simulink model "UAVIntegratedNavigationSystem"  (R2020b)
settings: Solver=FixedStepAuto  StartTime=0.0  StopTime=TFinal  FixedStep=IMUtime  RelTol=1e-3
values from neighbouring files (symbols this model uses):
  AIONtime = 1    [ModelSettings.m]
  BiasAccel = 9.81E-4    (= 0.000981)    [ModelSettings.m]
  BiasGyro = 2.424068405548E-4    (= 0.000242406840555)    [ModelSettings.m]
  CorrTimeOrientationGNSS = 1    [ModelSettings.m]
  CorrTimePositionGNSS = 1    [ModelSettings.m]
  CorrTimeVelocityGNSS = 1    [ModelSettings.m]
  delay = 1.5    [ModelSettings.m]
  e = 0.081819106    [ModelSettings.m]
  g0 = 9.780327    [ModelSettings.m]
  GNSStime = 0.2    [ModelSettings.m]
  H0 = 0.1    [ModelSettings.m]
  IMUtime = 0.01    [ModelSettings.m]
  indUAV = 2    [ModelSettings.m]
  LambdaInit = 0.6555    [ModelSettings.m]
  mass = 0.7    [ModelSettings.m]
  N = 100    [ModelSettings.m]
  PhiInit = 0.968    [ModelSettings.m]
  PitchDown = -PitchUp    (= -0.1)    [ModelSettings.m]
  PitchUp = 0.1    [ModelSettings.m]
  Ra = 6378.245    [ModelSettings.m]
  RollDown = -RollUp    (= -0.1)    [ModelSettings.m]
  RollUp = 0.1    [ModelSettings.m]
  SigmaAccel = 9.81E-4    (= 0.000981)    [ModelSettings.m]
  SigmaAION = 30    [ModelSettings.m]
  SigmaAltitudeGNSS = 3    [ModelSettings.m]
  SigmaGyro = 2.666475246102E-6    (= 2.6664752461e-06)    [ModelSettings.m]
  SigmaLaser = 5    [ModelSettings.m]
  SigmaOrientationGNSS = 0.00349    [ModelSettings.m]
  SigmaPositionGNSS = 1.5    [ModelSettings.m]
  SigmaVelocityGNSS = 0.03    [ModelSettings.m]
  SigmaVelocityUpGNSS = 0.03    [ModelSettings.m]
  U1down = 0    [ModelSettings.m]
  U1up = 4 * ForceCoeff * OmegaMax^2    (= 9.9858124)    [ModelSettings.m]
  U2down = -U2up    (= -2.4964531)    [ModelSettings.m]
  U2up = ForceCoeff * OmegaMax^2    (= 2.4964531)    [ModelSettings.m]
  U3down = -U3up    (= -2.4964531)    [ModelSettings.m]
  U3up = ForceCoeff * OmegaMax^2    (= 2.4964531)    [ModelSettings.m]
  U4down = -U4up    (= -0.2494604)    [ModelSettings.m]
  U4up = 2 * DragCoeff * OmegaMax^2    (= 0.2494604)    [ModelSettings.m]
  WEarth = 7.2921158553E-5    (= 7.2921158553e-05)    [ModelSettings.m]
undefined symbols (not defined in the file or in its folder): deg, Newton, rad, Raphson, s
libraries: simulink x11, sharedtransform x7, pid_lib x6, aerolibconvert2 x4, sharedutil x4
(part 4 of 5)

== system UAVIntegratedNavigationSystem/Блок модели динамики квадрокоптера + САУ/Полетный контроллер/Удержание положения/Row 1 ==
  Psi : Inport
  "R [1, 1]" : Subsystem
  "R [1, 2]" : Subsystem
  "R[1, 1]" : Outport
  "R[1, 2]" : Outport  Port=2
  wires:
  Psi/1 -> "R [1, 1]"/1(" Psi"), "R [1, 2]"/1(" Psi")
  "R [1, 1]"/1(R[1,1]) -> "R[1, 1]"/1
  "R [1, 2]"/1(R[1,2]) -> "R[1, 2]"/1

== system UAVIntegratedNavigationSystem/Блок модели динамики квадрокоптера + САУ/Полетный контроллер/Удержание положения/Row 2 ==
  Psi : Inport
  "R [2, 1]" : Subsystem
  "R [2, 2]" : Subsystem
  "R[2, 1]" : Outport
  "R[2, 2]" : Outport  Port=2
  wires:
  "R [2, 1]"/1(R[2,1]) -> "R[2, 1]"/1
  "R [2, 2]"/1(R[2,2]) -> "R[2, 2]"/1
  Psi/1 -> "R [2, 1]"/1(" Psi"), "R [2, 2]"/1(" Psi")

== system UAVIntegratedNavigationSystem/Блок модели динамики квадрокоптера + САУ/Упрощенная динамика БЛА /Векторы ускорений действующих сил/Ускорение силы гравитации ==
  g : Inport
  "(X, Y, Z, phi)" : Inport  Port=2
  3x3 Cross Product : sharedutil/3x3 Cross Product  aMode=aMode
      settings: SourceProductBaseCode=AE,PW,MT,UV,VE,VP
  3x3 Cross Product1 : sharedutil/3x3 Cross Product  aMode=aMode
      settings: SourceProductBaseCode=AE,PW,MT,UV,VE,VP
  Add : Sum  Inputs=+-
  Bus Selector : BusSelector  OutputSignals=X,Y,Z,phi
  Constant : Constant  Value=0
  Constant1 : Constant  Value=0
  Constant5 : Constant  Value=0
  Cos : Trigonometry  Operator=cos
  Gain : Gain  Gain=-1
  Mux : Mux  Inputs=3
  Mux1 : Mux  Inputs=3
  Mux2 : Mux  Inputs=3
  Sin2 : Trigonometry
  WEarth : Gain  Gain=WEarth
  WEarth1 : Gain  Gain=WEarth
  Вектор ускорения силы гравитации : Outport
  wires:
  Constant/1 -> Mux/1
  Constant1/1 -> Mux/3
  Gain/1 -> Mux/2
  g/1 -> Gain/1
  3x3 Cross Product/1 -> 3x3 Cross Product1/2
  Mux2/1 -> 3x3 Cross Product/2
  WEarth1/1 -> Mux1/2
  Constant5/1 -> Mux1/3
  Cos/1 -> WEarth/1
  WEarth/1 -> Mux1/1
  Sin2/1 -> WEarth1/1
  Mux1/1 -> 3x3 Cross Product1/1, 3x3 Cross Product/1
  Bus Selector/4 -> Sin2/1, Cos/1  "<phi>"
  "(X, Y, Z, phi)"/1 -> Bus Selector/1
  Mux/1 -> Add/1
  Add/1 -> Вектор ускорения силы гравитации/1
  Bus Selector/2 -> Mux2/2  "<Y>"
  Bus Selector/1 -> Mux2/1  "<X>"
  Bus Selector/3 -> Mux2/3  "<Z>"
  3x3 Cross Product1/1 -> Add/2  "Переносное ускорение"

== system UAVIntegratedNavigationSystem/Блок модели динамики квадрокоптера + САУ/Упрощенная динамика БЛА /Векторы ускорений действующих сил/Ускорение силы тяги ==
  U1 : Inport
  Pitch : Inport  Port=2
  Roll : Inport  Port=3
  Psi : Inport  Port=4
  1 / m : Gain  Gain=1/ mass
  Mux : Mux  Inputs=3
  ThrustAccX : Subsystem
  ThrustAccY : Subsystem
  ThrustAccZ : Subsystem
  Вектор ускорения силы тяги : Outport
  wires:
  U1/1 -> 1 / m/1
  Psi/1 -> ThrustAccX/4(Psi), ThrustAccZ/3(Psi)
  Pitch/1 -> ThrustAccX/2(Pitch), ThrustAccY/2(Pitch), ThrustAccZ/1(Pitch)
  1 / m/1 -> ThrustAccY/1(U1 / m), ThrustAccZ/4(U1 / m), ThrustAccX/1(U1 / m)
  Roll/1 -> ThrustAccZ/2(Roll), ThrustAccY/3(Roll), ThrustAccX/3(Roll)
  ThrustAccX/1(ThrustAccX) -> Mux/1
  ThrustAccY/1(ThrustAccY) -> Mux/2
  ThrustAccZ/1(ThrustAccZ) -> Mux/3
  Mux/1 -> Вектор ускорения силы тяги/1

== system UAVIntegratedNavigationSystem/Блок модели динамики квадрокоптера + САУ/Упрощенная динамика БЛА /Простр. движение Ц.М. БПЛА (Геогр. СК)/Координаты БПЛА (Географ. СК) ==
  Velocity : Inport
  R : Inport  Port=2
  "Север(0), Восток(0)" : Inport  Port=3
  Bus Creator : BusCreator  Inputs=5
  Demux : Demux  Outputs=2
  Demux1 : Demux  Outputs=3
  Demux2 : Demux  Outputs=2
  Integrator : Integrator  InitialCondition=PhiInit
  Integrator1 : Integrator  InitialConditionSource=external
  Integrator2 : Integrator
  Integrator3 : Integrator  InitialConditionSource=external
  Integrator4 : Integrator  InitialCondition=LambdaInit
  Product : Product
  Trigonometric Function : Trigonometry  Operator=cos
  dLambda/dt : Product  Inputs=*/
  dPhi/dt : Product  Inputs=*/
  "Coord, phi, lambda" : Outport
  wires:
  R/1 -> Demux/1
  dPhi/dt/1 -> Integrator/1
  Demux/1 -> dPhi/dt/2
  Velocity/1 -> Demux1/1
  Demux1/1 -> dPhi/dt/1, Integrator1/1
  Demux/2 -> Product/2
  Integrator1/1 -> Bus Creator/1  "X"
  Integrator2/1 -> Bus Creator/2  "Y"
  Integrator3/1 -> Bus Creator/3  "Z"
  Demux1/2 -> Integrator2/1
  Demux1/3 -> dLambda/dt/1, Integrator3/1
  Integrator/1 -> Bus Creator/4, Trigonometric Function/1  "phi"
  Trigonometric Function/1 -> Product/1
  Product/1 -> dLambda/dt/2
  dLambda/dt/1 -> Integrator4/1
  Integrator4/1 -> Bus Creator/5  "lambda"
  Bus Creator/1 -> "Coord, phi, lambda"/1
  "Север(0), Восток(0)"/1 -> Demux2/1
  Demux2/1 -> Integrator1/2
  Demux2/2 -> Integrator3/2

== system UAVIntegratedNavigationSystem/Блок модели динамики квадрокоптера + САУ/Упрощенная динамика БЛА /Простр. движение Ц.М. БПЛА (Геогр. СК)/Радиус - вектор точки местоположения Ц.М. БПЛА (phi) ==
  Phi : Inport
  Add2 : Sum  Inputs=+-
  Add3 : Sum  Inputs=+-
  Add4 : Sum
  Add5 : Sum
  Constant2 : Constant  Value=Ra
  Constant3 : Constant  Value=H0
  Constant4 : Constant
  Constant5 : Constant  Value=1.5
  Divide : Product  Inputs=*/
  Divide1 : Product  Inputs=*/
  Mux : Mux  Inputs=2
  Power : Math  Operator=pow  SaturateOnIntegerOverflow=on
  Product1 : Product
  Product2 : Product
  Sin1 : Trigonometry
  Sqrt : Sqrt  SaturateOnIntegerOverflow=on
  Square2 : Math  Operator=square  SaturateOnIntegerOverflow=on
  Square3 : Math  Operator=square  SaturateOnIntegerOverflow=on
  e1 : Constant  Value=e
  "km -> m" : Gain  Gain=1000
  "km -> m 1" : Gain  Gain=1000
  "R, м" : Outport
  wires:
  Phi/1 -> Sin1/1
  Constant2/1 -> "km -> m"/1
  Constant3/1 -> "km -> m 1"/1
  e1/1 -> Square2/1
  Square2/1 -> Product2/1, Add2/2
  Constant4/1 -> Add2/1, Add3/1
  "km -> m"/1 -> Product1/1, Divide1/1
  Add2/1 -> Product1/2
  Sin1/1 -> Square3/1
  Square3/1 -> Product2/2
  Product2/1 -> Add3/2
  Product1/1 -> Divide/1
  Divide/1 -> Add4/1
  "km -> m 1"/1 -> Add5/1, Add4/2
  Add4/1 -> Mux/1  "R1"
  Add3/1 -> Power/1, Sqrt/1
  Power/1 -> Divide/2
  Constant5/1 -> Power/2
  Mux/1 -> "R, м"/1
  Sqrt/1 -> Divide1/2
  Divide1/1 -> Add5/2
  Add5/1 -> Mux/2  "R2"

== system UAVIntegratedNavigationSystem/Блок модели динамики квадрокоптера + САУ/Упрощенная динамика БЛА /Простр. движение Ц.М. БПЛА (Геогр. СК)/Скорости БПЛА (Географ. СК) ==
  AccX : Inport
  AccY : Inport  Port=2
  AccZ : Inport  Port=3
  R : Inport  Port=4
  phi : Inport  Port=5
  Integrator : Integrator
  Integrator1 : Integrator
  Integrator2 : Integrator
  Mux : Mux  Inputs=3
  Mux1 : Mux  Inputs=3
  Mux2 : Mux  Inputs=3
  Mux3 : Mux  Inputs=2
  dVx / dt : Subsystem
  dVy / dt : Subsystem
  dVz / dt : Subsystem
  Velocity : Outport
  Относ и Кориолис ускорение : Outport  Port=2
  wires:
  Integrator/1 -> dVz / dt/5(Vx), dVy / dt/4(Vx), dVx / dt/5(Vx), Mux/1
  Integrator1/1 -> dVz / dt/3(Vy), dVx / dt/3(Vy), Mux/2
  Integrator2/1 -> Mux/3, dVz / dt/4(Vz), dVx / dt/4(Vz), dVy / dt/3(Vz)
  AccX/1 -> dVx / dt/1(AccX)
  R/1 -> dVx / dt/2(R), dVz / dt/2(R), dVy / dt/2(R)
  dVx / dt/1(dVx/dt) -> Integrator/1
  AccY/1 -> dVy / dt/1(AccY)
  dVy / dt/1(dVy/dt) -> Integrator1/1
  AccZ/1 -> dVz / dt/1(AccZ)
  dVz / dt/1(dVz/dt) -> Integrator2/1
  Mux/1 -> Velocity/1
  phi/1 -> dVx / dt/6(phi), dVy / dt/5(phi), dVz / dt/6(phi)
  dVx / dt/2(AccX относ) -> Mux1/1
  dVy / dt/2(AccY относ) -> Mux1/2
  dVz / dt/2(AccZ относ) -> Mux1/3
  dVx / dt/3(AccX кориолис) -> Mux2/1
  dVy / dt/3(AccY кориолис) -> Mux2/2
  dVz / dt/3(AccZ кориолис) -> Mux2/3
  Mux1/1 -> Mux3/1
  Mux2/1 -> Mux3/2
  Mux3/1 -> Относ и Кориолис ускорение/1

== system UAVIntegratedNavigationSystem/Блок модели динамики квадрокоптера + САУ/Упрощенная динамика БЛА /Решение уравнения Пуассона/ДУ кватернион ==
  note: p q r Q0 Q1 Q2 Q3
  state : Inport
  Bus Creator : BusCreator  Inputs=3
  Bus Selector : BusSelector  OutputSignals=wx,wy,wz
  Bus Selector1 : BusSelector  OutputSignals=wz,wy,wx
  Bus Selector2 : BusSelector  OutputSignals=wy,wz,wx
  Bus Selector3 : BusSelector  OutputSignals=wx,wz,wy
  Constant : Constant  Value=0
  Demux : Demux  Outputs=[1 1 1 4]
      settings: DisplayOption=none
  Dot Product {1..4} (4 alike) : DotProduct  InputSameDT=on  OutDataTypeStr=Inherit: Inherit via internal rule
  Gain {1..6} (6 alike) : Gain  Gain=-1  SaturateOnIntegerOverflow=on  OutDataTypeStr=Inherit: Same as input  ParamDataTypeStr=Inherit: Same as input
  Gain 7 : Gain  Gain=0.5  SaturateOnIntegerOverflow=on  OutDataTypeStr=Inherit: Same as input  ParamDataTypeStr=Inherit: Same as input
  Mux{1..4,6} (5 alike) : Mux
  d(Q)/dt : Outport
  wires:
  Mux6/1 -> Gain 7/1
  state/1 -> Demux/1
  Gain 2/1 -> Mux2/4
  Bus Selector/1 -> Gain 4/1  "<wx>"
  Mux2/1 -> Dot Product 1/2
  Mux3/1 -> Dot Product 2/2
  Mux4/1 -> Dot Product 3/2
  Demux/1 -> Bus Creator/1  "wx"
  Demux/2 -> Bus Creator/2  "wy"
  Demux/3 -> Bus Creator/3  "wz"
  Gain 5/1 -> Mux4/2
  Gain 3/1 -> Mux3/3
  Mux1/1 -> Dot Product 4/2
  Bus Creator/1 -> Bus Selector2/1, Bus Selector1/1, Bus Selector/1, Bus Selector3/1
  Constant/1 -> Mux2/1, Mux1/2, Mux3/4, Mux4/3
  Bus Selector3/3 -> Gain 1/1  "<wy>"
  Gain 4/1 -> Mux2/2
  Gain 6/1 -> Mux2/3
  Bus Selector/2 -> Gain 6/1  "<wy>"
  Bus Selector/3 -> Gain 2/1  "<wz>"
  Dot Product 2/1 -> Mux6/4
  Dot Product 3/1 -> Mux6/3
  Dot Product 4/1 -> Mux6/2
  Dot Product 1/1 -> Mux6/1
  Demux/4 -> Dot Product 3/1, Dot Product 4/1, Dot Product 1/1, Dot Product 2/1
  Gain 7/1 -> d(Q)/dt/1
  Bus Selector3/1 -> Mux1/1  "<wx>"
  Bus Selector3/2 -> Mux1/3  "<wz>"
  Gain 1/1 -> Mux1/4
  Bus Selector1/3 -> Gain 3/1  "<wx>"
  Bus Selector1/2 -> Mux3/2  "<wy>"
  Bus Selector1/1 -> Mux3/1  "<wz>"
  Bus Selector2/1 -> Mux4/1  "<wy>"
  Bus Selector2/2 -> Gain 5/1  "<wz>"
  Bus Selector2/3 -> Mux4/4  "<wx>"

== system UAVIntegratedNavigationSystem/Блок модели динамики квадрокоптера + САУ/Упрощенная динамика БЛА /Решение уравнения Пуассона/Нормирование кватерниона ==
  q : Inport  PortDimensions=4
  Product : Product  Inputs=*/  InputSameDT=on  RndMeth=Zero  SaturateOnIntegerOverflow=on  OutDataTypeStr=Inherit: Same as first input
  Square : Math  Operator=square  SignedPower=on  SaturateOnIntegerOverflow=on
  Square Root : Sqrt  Operator=signedSqrt  AlgorithmType=Newton-Raphson  SaturateOnIntegerOverflow=on
  Sum : Sum  Inputs=1  InputSameDT=on  SaturateOnIntegerOverflow=on  OutDataTypeStr=Inherit: Same as first input
  qnorm : Outport  PortDimensions=4
  wires:
  Product/1 -> qnorm/1
  Square Root/1 -> Product/2
  Square/1 -> Sum/1
  Sum/1 -> Square Root/1
  q/1 -> Product/1, Square/1

== system UAVIntegratedNavigationSystem/Показания АИОН + ЛД/Измерения АИОН + ЛД/Вектор случайных аддитивных ошибок в определении высоты местоположения БЛА/ФФ  ==
  Band-Limited White Noise1 : simulink/Sources/Band-Limited White Noise  Cov=[AIONtime]  Ts=AIONtime  seed=[23341]
  "sigma " : Gain  Gain=SigmaLaser
  Случ. погрешность ЛД по высоте : Outport
  wires:
  Band-Limited White Noise1/1 -> "sigma "/1
  "sigma "/1 -> Случ. погрешность ЛД по высоте/1

== system UAVIntegratedNavigationSystem/Показания АИОН + ЛД/Измерения АИОН + ЛД/Вектор случайных аддитивных ошибок в определении координат местоположения БЛА/ФФ  ==
  Band-Limited White Noise1 : simulink/Sources/Band-Limited White Noise  Cov=[AIONtime]  Ts=AIONtime  seed=[23341]
  sigma : Gain  Gain=SigmaAION
  Случ. погрешность АИОНпо координатам : Outport
  wires:
  sigma/1 -> Случ. погрешность АИОНпо координатам/1
  Band-Limited White Noise1/1 -> sigma/1

== system UAVIntegratedNavigationSystem/Показания приемника ГНСС/Измерения ГНСС/Вектор случайных аддитивных ошибок в определении координат местопложения БЛА/ФФ  ==
  - 1 / CorrTime : Gain  Gain=-1 / CorrTimePositionGNSS
  Add : Sum
  Band-Limited White Noise1 : simulink/Sources/Band-Limited White Noise  Cov=[GNSStime]  Ts=GNSStime  seed=[23341]
  Integrator2 : Integrator  InitialCondition=0.001
  sigma * sqrt(2 / CorrTime) : Gain  Gain=SigmaPositionGNSS * sqrt(2 / CorrTimePositionGNSS)
  Случ. погрешность ГНСС по координатам : Outport
  wires:
  Integrator2/1 -> - 1 / CorrTime/1, Случ. погрешность ГНСС по координатам/1
  Band-Limited White Noise1/1 -> sigma * sqrt(2 / CorrTime)/1
  Add/1 -> Integrator2/1
  - 1 / CorrTime/1 -> Add/1
  sigma * sqrt(2 / CorrTime)/1 -> Add/2

== system UAVIntegratedNavigationSystem/Показания приемника ГНСС/Измерения ГНСС/Вектор случайных аддитивных ошибок в определении координат местопложения БЛА/ФФ 1 ==
  - 1 / CorrTime : Gain  Gain=-1 / CorrTimePositionGNSS
  Add : Sum
  Band-Limited White Noise1 : simulink/Sources/Band-Limited White Noise  Cov=[GNSStime]  Ts=GNSStime  seed=[23341]
  Integrator2 : Integrator  InitialCondition=0.001
  sigma * sqrt(2 / CorrTime) : Gain  Gain=SigmaAltitudeGNSS * sqrt(2 / CorrTimePositionGNSS)
  Случ. погрешность ГНСС по высоте : Outport
  wires:
  Add/1 -> Integrator2/1
  Integrator2/1 -> Случ. погрешность ГНСС по высоте/1, - 1 / CorrTime/1
  sigma * sqrt(2 / CorrTime)/1 -> Add/2
  - 1 / CorrTime/1 -> Add/1
  Band-Limited White Noise1/1 -> sigma * sqrt(2 / CorrTime)/1

== system UAVIntegratedNavigationSystem/Показания приемника ГНСС/Измерения ГНСС/Вектор случайных аддитивных ошибок в определении ориентации БЛА/ФФ  ==
  - 1 / CorrTime : Gain  Gain=-1 / CorrTimeOrientationGNSS
  Add : Sum
  Band-Limited White Noise1 : simulink/Sources/Band-Limited White Noise  Cov=[GNSStime]  Ts=GNSStime  seed=[23341]
  Integrator2 : Integrator  InitialCondition=0.001
  sigma * sqrt(2 / CorrTime) : Gain  Gain=SigmaOrientationGNSS * sqrt(2 / CorrTimeOrientationGNSS)
  Случ. погрешность ГНСС по углам : Outport
  wires:
  Integrator2/1 -> - 1 / CorrTime/1, Случ. погрешность ГНСС по углам/1
  Band-Limited White Noise1/1 -> sigma * sqrt(2 / CorrTime)/1
  Add/1 -> Integrator2/1
  - 1 / CorrTime/1 -> Add/1
  sigma * sqrt(2 / CorrTime)/1 -> Add/2

== system UAVIntegratedNavigationSystem/Показания приемника ГНСС/Измерения ГНСС/Вектор случайных аддитивных ошибок в определении проекций скорости  БЛА/ФФ  ==
  - 1 / CorrTime : Gain  Gain=-1 / CorrTimeVelocityGNSS
  Add : Sum
  Band-Limited White Noise1 : simulink/Sources/Band-Limited White Noise  Cov=[GNSStime]  Ts=GNSStime  seed=[23341]
  Integrator2 : Integrator  InitialCondition=0.001
  sigma * sqrt(2 / CorrTime) : Gain  Gain=SigmaVelocityGNSS * sqrt(2 / CorrTimeVelocityGNSS)
  Случ. погрешность ГНСС по скоростям : Outport
  wires:
  Integrator2/1 -> - 1 / CorrTime/1, Случ. погрешность ГНСС по скоростям/1
  Band-Limited White Noise1/1 -> sigma * sqrt(2 / CorrTime)/1
  Add/1 -> Integrator2/1
  - 1 / CorrTime/1 -> Add/1
  sigma * sqrt(2 / CorrTime)/1 -> Add/2

== system UAVIntegratedNavigationSystem/Показания приемника ГНСС/Измерения ГНСС/Вектор случайных аддитивных ошибок в определении проекций скорости  БЛА/ФФ 1 ==
  - 1 / CorrTime : Gain  Gain=-1 / CorrTimeVelocityGNSS
  Add : Sum
  Band-Limited White Noise1 : simulink/Sources/Band-Limited White Noise  Cov=[GNSStime]  Ts=GNSStime  seed=[23341]
  Integrator2 : Integrator  InitialCondition=0.001
  sigma * sqrt(2 / CorrTime) : Gain  Gain=SigmaVelocityUpGNSS * sqrt(2 / CorrTimeVelocityGNSS)
  Случ. погрешность ГНСС по скоростям : Outport
  wires:
  Add/1 -> Integrator2/1
  Integrator2/1 -> Случ. погрешность ГНСС по скоростям/1, - 1 / CorrTime/1
  sigma * sqrt(2 / CorrTime)/1 -> Add/2
  - 1 / CorrTime/1 -> Add/1
  Band-Limited White Noise1/1 -> sigma * sqrt(2 / CorrTime)/1

== system UAVIntegratedNavigationSystem/Алгоритм ИНС /Алгоритм Навигации/Скорости БПЛА (Географ. СК)/dVx // dt/AccX Кориолис ==
  VelZ : Inport
  phi : Inport  Port=2
  2 : Constant  Value=2
  Gain : Gain  Gain=-1
  Product : Product  Inputs=4
  Trigonometric Function : Trigonometry
  WEarth : Constant  Value=WEarth
  AccX Кориолис : Outport
  wires:
  Trigonometric Function/1 -> Product/1
  Product/1 -> Gain/1
  WEarth/1 -> Product/2
  2/1 -> Product/4
  phi/1 -> Trigonometric Function/1
  VelZ/1 -> Product/3
  Gain/1 -> AccX Кориолис/1

== system UAVIntegratedNavigationSystem/Алгоритм ИНС /Алгоритм Навигации/Скорости БПЛА (Географ. СК)/dVx // dt/AccX Относительное ==
  VelX : Inport
  VelY : Inport  Port=2
  VelZ : Inport  Port=3
  R : Inport  Port=4
  phi : Inport  Port=5
  Add : Sum  Inputs=--
  Demux : Demux  Outputs=2
  Divide : Product  Inputs=*/
  Divide1 : Product  Inputs=*/
  Product1 : Product
  Product2 : Product
  Product3 : Product
  Trigonometric Function1 : Trigonometry  Operator=tan
  AccX Относительное : Outport
  wires:
  R/1 -> Demux/1
  VelZ/1 -> Product2/2, Product2/1
  Demux/2 -> Divide1/2  "R2"
  Trigonometric Function1/1 -> Product3/2
  Divide1/1 -> Product3/1
  Product2/1 -> Divide1/1
  phi/1 -> Trigonometric Function1/1
  Product3/1 -> Add/1
  Add/1 -> AccX Относительное/1
  Demux/1 -> Divide/2  "R1"
  Product1/1 -> Divide/1
  VelX/1 -> Product1/1
  VelY/1 -> Product1/2
  Divide/1 -> Add/2

== system UAVIntegratedNavigationSystem/Алгоритм ИНС /Алгоритм Навигации/Скорости БПЛА (Географ. СК)/dVy // dt/AccY Кориолис ==
  VelZ : Inport
  phi : Inport  Port=2
  2 : Constant  Value=2
  Product : Product  Inputs=4
  Trigonometric Function : Trigonometry  Operator=cos
  WEarth : Constant  Value=WEarth
  AccX Кориолис : Outport
  wires:
  Trigonometric Function/1 -> Product/1
  WEarth/1 -> Product/2
  2/1 -> Product/4
  phi/1 -> Trigonometric Function/1
  VelZ/1 -> Product/3
  Product/1 -> AccX Кориолис/1

== system UAVIntegratedNavigationSystem/Алгоритм ИНС /Алгоритм Навигации/Скорости БПЛА (Географ. СК)/dVy // dt/AccY Относительное ==
  VelX : Inport
  VelZ : Inport  Port=2
  R : Inport  Port=3
  phi : Inport  Port=4
  Add : Sum  Inputs=+-
  Demux : Demux  Outputs=2
  Divide : Product  Inputs=*/
  Divide1 : Product  Inputs=*/
  Product1 : Product
  Product2 : Product
  Product3 : Product
  Trigonometric Function1 : Trigonometry  Operator=tan
  AccY Относительное : Outport
  wires:
  R/1 -> Demux/1
  VelZ/1 -> Product2/2, Product2/1
  Product2/1 -> Divide1/1
  phi/1 -> Trigonometric Function1/1
  Divide1/1 -> Add/1
  Add/1 -> AccY Относительное/1
  Product1/1 -> Divide/1
  VelX/1 -> Product1/2, Product1/1
  Divide/1 -> Product3/1
  Demux/2 -> Divide/2  "R2"
  Demux/1 -> Divide1/2  "R1"
  Product3/1 -> Add/2
  Trigonometric Function1/1 -> Product3/2

== system UAVIntegratedNavigationSystem/Алгоритм ИНС /Алгоритм Навигации/Скорости БПЛА (Географ. СК)/dVz // dt/AccZ Кориолис ==
  VelX : Inport
  VelY : Inport  Port=2
  phi : Inport  Port=3
  2 : Constant  Value=2
  Add1 : Sum  Inputs=+-
  Gain : Gain  Gain=-1
  Product : Product  Inputs=3
  Product4 : Product
  Product5 : Product
  Trigonometric Function2 : Trigonometry  Operator=cos
  Trigonometric Function3 : Trigonometry
  WEarth : Constant  Value=WEarth
  AccZ Кориолис : Outport
  wires:
  Product5/1 -> Add1/2
  Add1/1 -> Product/3
  Product4/1 -> Add1/1
  2/1 -> Product/1
  Trigonometric Function2/1 -> Product4/2
  Trigonometric Function3/1 -> Product5/2
  WEarth/1 -> Product/2
  phi/1 -> Trigonometric Function2/1, Trigonometric Function3/1
  Product/1 -> Gain/1
  Gain/1 -> AccZ Кориолис/1
  VelY/1 -> Product4/1
  VelX/1 -> Product5/1

== system UAVIntegratedNavigationSystem/Алгоритм ИНС /Алгоритм Навигации/Скорости БПЛА (Географ. СК)/dVz // dt/AccZ Относительное ==
  VelX : Inport
  VelY : Inport  Port=2
  VelZ : Inport  Port=3
  R : Inport  Port=4
  phi : Inport  Port=5
  Add : Sum  Inputs=+-
  Demux : Demux  Outputs=2
  Divide : Product  Inputs=*/
  Divide1 : Product  Inputs=*/
  Product1 : Product
  Product2 : Product
  Product3 : Product
  Trigonometric Function1 : Trigonometry  Operator=tan
  AccZ Относительное : Outport
  wires:
  R/1 -> Demux/1
  Demux/2 -> Divide1/2  "R2"
  Trigonometric Function1/1 -> Product3/2
  Divide1/1 -> Product3/1
  Product2/1 -> Divide1/1
  phi/1 -> Trigonometric Function1/1
  Product3/1 -> Add/1
  Add/1 -> AccZ Относительное/1
  Demux/1 -> Divide/2  "R1"
  Product1/1 -> Divide/1
  Divide/1 -> Add/2
  VelY/1 -> Product1/1
  VelZ/1 -> Product2/2, Product1/2
  VelX/1 -> Product2/1

== system UAVIntegratedNavigationSystem/Алгоритм ИНС (коррекия БЧЭ)/Алгоритм Навигации/Скорости БПЛА (Географ. СК)/dVx // dt/AccX Кориолис ==
  VelZ : Inport
  phi : Inport  Port=2
  2 : Constant  Value=2
  Gain : Gain  Gain=-1
  Product : Product  Inputs=4
  Trigonometric Function : Trigonometry
  WEarth : Constant  Value=WEarth
  AccX Кориолис : Outport
  wires:
  Trigonometric Function/1 -> Product/1
  Product/1 -> Gain/1
  WEarth/1 -> Product/2
  2/1 -> Product/4
  phi/1 -> Trigonometric Function/1
  VelZ/1 -> Product/3
  Gain/1 -> AccX Кориолис/1

== system UAVIntegratedNavigationSystem/Алгоритм ИНС (коррекия БЧЭ)/Алгоритм Навигации/Скорости БПЛА (Географ. СК)/dVx // dt/AccX Относительное ==
  VelX : Inport
  VelY : Inport  Port=2
  VelZ : Inport  Port=3
  R : Inport  Port=4
  phi : Inport  Port=5
  Add : Sum  Inputs=--
  Demux : Demux  Outputs=2
  Divide : Product  Inputs=*/
  Divide1 : Product  Inputs=*/
  Product1 : Product
  Product2 : Product
  Product3 : Product
  Trigonometric Function1 : Trigonometry  Operator=tan
  AccX Относительное : Outport
  wires:
  R/1 -> Demux/1
  VelZ/1 -> Product2/2, Product2/1
  Demux/2 -> Divide1/2  "R2"
  Trigonometric Function1/1 -> Product3/2
  Divide1/1 -> Product3/1
  Product2/1 -> Divide1/1
  phi/1 -> Trigonometric Function1/1
  Product3/1 -> Add/1
  Add/1 -> AccX Относительное/1
  Demux/1 -> Divide/2  "R1"
  Product1/1 -> Divide/1
  VelX/1 -> Product1/1
  VelY/1 -> Product1/2
  Divide/1 -> Add/2

== system UAVIntegratedNavigationSystem/Алгоритм ИНС (коррекия БЧЭ)/Алгоритм Навигации/Скорости БПЛА (Географ. СК)/dVy // dt/AccY Кориолис ==
  VelZ : Inport
  phi : Inport  Port=2
  2 : Constant  Value=2
  Product : Product  Inputs=4
  Trigonometric Function : Trigonometry  Operator=cos
  WEarth : Constant  Value=WEarth
  AccX Кориолис : Outport
  wires:
  Trigonometric Function/1 -> Product/1
  WEarth/1 -> Product/2
  2/1 -> Product/4
  phi/1 -> Trigonometric Function/1
  VelZ/1 -> Product/3
  Product/1 -> AccX Кориолис/1

== system UAVIntegratedNavigationSystem/Алгоритм ИНС (коррекия БЧЭ)/Алгоритм Навигации/Скорости БПЛА (Географ. СК)/dVy // dt/AccY Относительное ==
  VelX : Inport
  VelZ : Inport  Port=2
  R : Inport  Port=3
  phi : Inport  Port=4
  Add : Sum  Inputs=+-
  Demux : Demux  Outputs=2
  Divide : Product  Inputs=*/
  Divide1 : Product  Inputs=*/
  Product1 : Product
  Product2 : Product
  Product3 : Product
  Trigonometric Function1 : Trigonometry  Operator=tan
  AccY Относительное : Outport
  wires:
  R/1 -> Demux/1
  VelZ/1 -> Product2/2, Product2/1
  Product2/1 -> Divide1/1
  phi/1 -> Trigonometric Function1/1
  Divide1/1 -> Add/1
  Add/1 -> AccY Относительное/1
  Product1/1 -> Divide/1
  VelX/1 -> Product1/2, Product1/1
  Divide/1 -> Product3/1
  Demux/2 -> Divide/2  "R2"
  Demux/1 -> Divide1/2  "R1"
  Product3/1 -> Add/2
  Trigonometric Function1/1 -> Product3/2

== system UAVIntegratedNavigationSystem/Алгоритм ИНС (коррекия БЧЭ)/Алгоритм Навигации/Скорости БПЛА (Географ. СК)/dVz // dt/AccZ Кориолис ==
  VelX : Inport
  VelY : Inport  Port=2
  phi : Inport  Port=3
  2 : Constant  Value=2
  Add1 : Sum  Inputs=+-
  Gain : Gain  Gain=-1
  Product : Product  Inputs=3
  Product4 : Product
  Product5 : Product
  Trigonometric Function2 : Trigonometry  Operator=cos
  Trigonometric Function3 : Trigonometry
  WEarth : Constant  Value=WEarth
  AccZ Кориолис : Outport
  wires:
  Product5/1 -> Add1/2
  Add1/1 -> Product/3
  Product4/1 -> Add1/1
  2/1 -> Product/1
  Trigonometric Function2/1 -> Product4/2
  Trigonometric Function3/1 -> Product5/2
  WEarth/1 -> Product/2
  phi/1 -> Trigonometric Function2/1, Trigonometric Function3/1
  Product/1 -> Gain/1
  Gain/1 -> AccZ Кориолис/1
  VelY/1 -> Product4/1
  VelX/1 -> Product5/1

== system UAVIntegratedNavigationSystem/Алгоритм ИНС (коррекия БЧЭ)/Алгоритм Навигации/Скорости БПЛА (Географ. СК)/dVz // dt/AccZ Относительное ==
  VelX : Inport
  VelY : Inport  Port=2
  VelZ : Inport  Port=3
  R : Inport  Port=4
  phi : Inport  Port=5
  Add : Sum  Inputs=+-
  Demux : Demux  Outputs=2
  Divide : Product  Inputs=*/
  Divide1 : Product  Inputs=*/
  Product1 : Product
  Product2 : Product
  Product3 : Product
  Trigonometric Function1 : Trigonometry  Operator=tan
  AccZ Относительное : Outport
  wires:
  R/1 -> Demux/1
  Demux/2 -> Divide1/2  "R2"
  Trigonometric Function1/1 -> Product3/2
  Divide1/1 -> Product3/1
  Product2/1 -> Divide1/1
  phi/1 -> Trigonometric Function1/1
  Product3/1 -> Add/1
  Add/1 -> AccZ Относительное/1
  Demux/1 -> Divide/2  "R1"
  Product1/1 -> Divide/1
  Divide/1 -> Add/2
  VelY/1 -> Product1/1
  VelZ/1 -> Product2/2, Product1/2
  VelX/1 -> Product2/1

== system UAVIntegratedNavigationSystem/Блок модели динамики квадрокоптера + САУ/Полетный контроллер/Удержание положения/Row 1/R [1, 1] ==
  " Psi" : Inport
  Cos psi 1 : Trigonometry
  R[1,1] : Outport
  wires:
  " Psi"/1 -> Cos psi 1/1
  Cos psi 1/1 -> R[1,1]/1

== system UAVIntegratedNavigationSystem/Блок модели динамики квадрокоптера + САУ/Полетный контроллер/Удержание положения/Row 1/R [1, 2] ==
  " Psi" : Inport
  Gain : Gain  Gain=-1
  Sin psi1 : Trigonometry  Operator=cos
  R[1,2] : Outport
  wires:
  " Psi"/1 -> Sin psi1/1
  Sin psi1/1 -> Gain/1
  Gain/1 -> R[1,2]/1

== system UAVIntegratedNavigationSystem/Блок модели динамики квадрокоптера + САУ/Полетный контроллер/Удержание положения/Row 2/R [2, 1] ==
  " Psi" : Inport
  Trigonometric Function : Trigonometry  Operator=cos
  R[2,1] : Outport
  wires:
  " Psi"/1 -> Trigonometric Function/1
  Trigonometric Function/1 -> R[2,1]/1

== system UAVIntegratedNavigationSystem/Блок модели динамики квадрокоптера + САУ/Полетный контроллер/Удержание положения/Row 2/R [2, 2] ==
  " Psi" : Inport
  Trigonometric Function : Trigonometry
  R[2,2] : Outport
  wires:
  " Psi"/1 -> Trigonometric Function/1
  Trigonometric Function/1 -> R[2,2]/1

== system UAVIntegratedNavigationSystem/Блок модели динамики квадрокоптера + САУ/Упрощенная динамика БЛА /Векторы ускорений действующих сил/Ускорение силы тяги/ThrustAccX ==
  U1 / m : Inport
  Pitch : Inport  Port=2
  Roll : Inport  Port=3
  Psi : Inport  Port=4
  Add : Sum  Inputs=-+
  Product : Product  Inputs=3
  Product1 : Product
  Product4 : Product
  Trigonometric Function1 : Trigonometry
  Trigonometric Function2 : Trigonometry  Operator=cos
  Trigonometric Function3 : Trigonometry  Operator=cos
  Trigonometric Function4 : Trigonometry
  Trigonometric Function5 : Trigonometry
  ThrustAccX : Outport
  wires:
  Trigonometric Function3/1 -> Product/3
  Trigonometric Function5/1 -> Product1/2
  Psi/1 -> Trigonometric Function3/1, Trigonometric Function4/1
  Trigonometric Function4/1 -> Product1/1
  Trigonometric Function2/1 -> Product/2
  Add/1 -> Product4/2
  Roll/1 -> Trigonometric Function5/1, Trigonometric Function2/1
  Product/1 -> Add/1
  Trigonometric Function1/1 -> Product/1
  Product1/1 -> Add/2
  Product4/1 -> ThrustAccX/1
  U1 / m/1 -> Product4/1
  Pitch/1 -> Trigonometric Function1/1

== system UAVIntegratedNavigationSystem/Блок модели динамики квадрокоптера + САУ/Упрощенная динамика БЛА /Векторы ускорений действующих сил/Ускорение силы тяги/ThrustAccY ==
  U1 / m : Inport
  Pitch : Inport  Port=2
  Roll : Inport  Port=3
  Product : Product
  Product1 : Product
  Trigonometric Function : Trigonometry  Operator=cos
  Trigonometric Function1 : Trigonometry  Operator=cos
  ThrustAccY : Outport
  wires:
  Trigonometric Function1/1 -> Product/2
  Pitch/1 -> Trigonometric Function/1
  Product/1 -> Product1/2
  Trigonometric Function/1 -> Product/1
  Roll/1 -> Trigonometric Function1/1
  U1 / m/1 -> Product1/1
  Product1/1 -> ThrustAccY/1

== system UAVIntegratedNavigationSystem/Блок модели динамики квадрокоптера + САУ/Упрощенная динамика БЛА /Векторы ускорений действующих сил/Ускорение силы тяги/ThrustAccZ ==
  Pitch : Inport
  Roll : Inport  Port=2
  Psi : Inport  Port=3
  U1 / m : Inport  Port=4
  Add : Sum
  Product1 : Product
  Product2 : Product  Inputs=3
  Product4 : Product
  Trigonometric Function1 : Trigonometry  Operator=cos
  Trigonometric Function2 : Trigonometry
  Trigonometric Function3 : Trigonometry
  Trigonometric Function4 : Trigonometry  Operator=cos
  Trigonometric Function5 : Trigonometry
  ThrustAccZ : Outport
  wires:
  Trigonometric Function3/1 -> Product2/3
  Trigonometric Function1/1 -> Product2/2
  Trigonometric Function4/1 -> Product1/1
  Product2/1 -> Add/1
  Product1/1 -> Add/2
  Trigonometric Function2/1 -> Product2/1
  Trigonometric Function5/1 -> Product1/2
  Add/1 -> Product4/1
  Pitch/1 -> Trigonometric Function2/1
  U1 / m/1 -> Product4/2
  Product4/1 -> ThrustAccZ/1
  Roll/1 -> Trigonometric Function1/1, Trigonometric Function5/1
  Psi/1 -> Trigonometric Function3/1, Trigonometric Function4/1

== system UAVIntegratedNavigationSystem/Блок модели динамики квадрокоптера + САУ/Упрощенная динамика БЛА /Простр. движение Ц.М. БПЛА (Геогр. СК)/Скорости БПЛА (Географ. СК)/dVx // dt ==
  AccX : Inport
  R : Inport  Port=2
  Vy : Inport  Port=3
  Vz : Inport  Port=4
  Vx : Inport  Port=5
  phi : Inport  Port=6
  AccX Кориолис : Subsystem
  AccX Относительное : Subsystem
  Add : Sum  Inputs=+++
  dVx/dt : Outport
  AccX относ : Outport  Port=2
  AccX кориолис : Outport  Port=3
  wires:
  AccX/1 -> Add/1
  Add/1 -> dVx/dt/1
  R/1 -> AccX Относительное/4(R)
  Vx/1 -> AccX Относительное/1(VelX)
  Vy/1 -> AccX Относительное/2(VelY)
  Vz/1 -> AccX Кориолис/1(VelZ), AccX Относительное/3(VelZ)
  phi/1 -> AccX Кориолис/2(phi), AccX Относительное/5(phi)
  AccX Относительное/1(AccX Относительное) -> AccX относ/1, Add/2
  AccX Кориолис/1(AccX Кориолис) -> AccX кориолис/1, Add/3

== system UAVIntegratedNavigationSystem/Блок модели динамики квадрокоптера + САУ/Упрощенная динамика БЛА /Простр. движение Ц.М. БПЛА (Геогр. СК)/Скорости БПЛА (Географ. СК)/dVy // dt ==
  AccY : Inport
  R : Inport  Port=2
  Vz : Inport  Port=3
  Vx : Inport  Port=4
  phi : Inport  Port=5
  AccY Кориолис : Subsystem
  AccY Относительное : Subsystem
  Add : Sum  Inputs=+++
  dVy/dt : Outport
  AccY относ : Outport  Port=2
  AccY кориолис : Outport  Port=3
  wires:
  AccY/1 -> Add/1
  Vx/1 -> AccY Относительное/1(VelX)
  R/1 -> AccY Относительное/3(R)
  Add/1 -> dVy/dt/1
  Vz/1 -> AccY Кориолис/1(VelZ), AccY Относительное/2(VelZ)
  phi/1 -> AccY Кориолис/2(phi), AccY Относительное/4(phi)
  AccY Кориолис/1(AccX Кориолис) -> Add/3, AccY кориолис/1
  AccY Относительное/1(AccY Относительное) -> AccY относ/1, Add/2

== system UAVIntegratedNavigationSystem/Блок модели динамики квадрокоптера + САУ/Упрощенная динамика БЛА /Простр. движение Ц.М. БПЛА (Геогр. СК)/Скорости БПЛА (Географ. СК)/dVz // dt ==
  AccZ : Inport
  R : Inport  Port=2
  Vy : Inport  Port=3
  Vz : Inport  Port=4
  Vx : Inport  Port=5
  phi : Inport  Port=6
  AccZ Кориолис : Subsystem
  AccZ Относительное : Subsystem
  Add : Sum  Inputs=+++
  dVz/dt : Outport
  AccZ относ : Outport  Port=2
  AccZ кориолис : Outport  Port=3
  wires:
  AccZ/1 -> Add/1
  Add/1 -> dVz/dt/1
  Vx/1 -> AccZ Относительное/1(VelX), AccZ Кориолис/1(VelX)
  Vy/1 -> AccZ Относительное/2(VelY), AccZ Кориолис/2(VelY)
  Vz/1 -> AccZ Относительное/3(VelZ)
  R/1 -> AccZ Относительное/4(R)
  phi/1 -> AccZ Кориолис/3(phi), AccZ Относительное/5(phi)
  AccZ Кориолис/1(AccZ Кориолис) -> AccZ кориолис/1, Add/3
  AccZ Относительное/1(AccZ Относительное) -> AccZ относ/1, Add/2

== system UAVIntegratedNavigationSystem/Блок модели динамики квадрокоптера + САУ/Упрощенная динамика БЛА /Простр. движение Ц.М. БПЛА (Геогр. СК)/Скорости БПЛА (Географ. СК)/dVx // dt/AccX Кориолис ==
  VelZ : Inport
  phi : Inport  Port=2
  2 : Constant  Value=2
  Gain : Gain  Gain=-1
  Product : Product  Inputs=4
  Trigonometric Function : Trigonometry
  WEarth : Constant  Value=WEarth
  AccX Кориолис : Outport
  wires:
  Trigonometric Function/1 -> Product/1
  Product/1 -> Gain/1
  WEarth/1 -> Product/2
  2/1 -> Product/4
  phi/1 -> Trigonometric Function/1
  VelZ/1 -> Product/3
  Gain/1 -> AccX Кориолис/1

== system UAVIntegratedNavigationSystem/Блок модели динамики квадрокоптера + САУ/Упрощенная динамика БЛА /Простр. движение Ц.М. БПЛА (Геогр. СК)/Скорости БПЛА (Географ. СК)/dVx // dt/AccX Относительное ==
  VelX : Inport
  VelY : Inport  Port=2
  VelZ : Inport  Port=3
  R : Inport  Port=4
  phi : Inport  Port=5
  Add : Sum  Inputs=--
  Demux : Demux  Outputs=2
  Divide : Product  Inputs=*/
  Divide1 : Product  Inputs=*/
  Product1 : Product
  Product2 : Product
  Product3 : Product
  Trigonometric Function1 : Trigonometry  Operator=tan
  AccX Относительное : Outport
  wires:
  R/1 -> Demux/1
  VelZ/1 -> Product2/2, Product2/1
  Demux/2 -> Divide1/2  "R2"
  Trigonometric Function1/1 -> Product3/2
  Divide1/1 -> Product3/1
  Product2/1 -> Divide1/1
  phi/1 -> Trigonometric Function1/1
  Product3/1 -> Add/1
  Add/1 -> AccX Относительное/1
  Demux/1 -> Divide/2  "R1"
  Product1/1 -> Divide/1
  VelX/1 -> Product1/1
  VelY/1 -> Product1/2
  Divide/1 -> Add/2

== system UAVIntegratedNavigationSystem/Блок модели динамики квадрокоптера + САУ/Упрощенная динамика БЛА /Простр. движение Ц.М. БПЛА (Геогр. СК)/Скорости БПЛА (Географ. СК)/dVy // dt/AccY Кориолис ==
  VelZ : Inport
  phi : Inport  Port=2
  2 : Constant  Value=2
  Product : Product  Inputs=4
  Trigonometric Function : Trigonometry  Operator=cos
  WEarth : Constant  Value=WEarth
  AccX Кориолис : Outport
  wires:
  Trigonometric Function/1 -> Product/1
  WEarth/1 -> Product/2
  2/1 -> Product/4
  phi/1 -> Trigonometric Function/1
  VelZ/1 -> Product/3
  Product/1 -> AccX Кориолис/1

== system UAVIntegratedNavigationSystem/Блок модели динамики квадрокоптера + САУ/Упрощенная динамика БЛА /Простр. движение Ц.М. БПЛА (Геогр. СК)/Скорости БПЛА (Географ. СК)/dVy // dt/AccY Относительное ==
  VelX : Inport
  VelZ : Inport  Port=2
  R : Inport  Port=3
  phi : Inport  Port=4
  Add : Sum  Inputs=+-
  Demux : Demux  Outputs=2
  Divide : Product  Inputs=*/
  Divide1 : Product  Inputs=*/
  Product1 : Product
  Product2 : Product
  Product3 : Product
  Trigonometric Function1 : Trigonometry  Operator=tan
  AccY Относительное : Outport
  wires:
  R/1 -> Demux/1
  VelZ/1 -> Product2/2, Product2/1
  Product2/1 -> Divide1/1
  phi/1 -> Trigonometric Function1/1
  Divide1/1 -> Add/1
  Add/1 -> AccY Относительное/1
  Product1/1 -> Divide/1
  VelX/1 -> Product1/2, Product1/1
  Divide/1 -> Product3/1
  Demux/2 -> Divide/2  "R2"
  Demux/1 -> Divide1/2  "R1"
  Product3/1 -> Add/2
  Trigonometric Function1/1 -> Product3/2

== system UAVIntegratedNavigationSystem/Блок модели динамики квадрокоптера + САУ/Упрощенная динамика БЛА /Простр. движение Ц.М. БПЛА (Геогр. СК)/Скорости БПЛА (Географ. СК)/dVz // dt/AccZ Кориолис ==
  VelX : Inport
  VelY : Inport  Port=2
  phi : Inport  Port=3
  2 : Constant  Value=2
  Add1 : Sum  Inputs=+-
  Gain : Gain  Gain=-1
  Product : Product  Inputs=3
  Product4 : Product
  Product5 : Product
  Trigonometric Function2 : Trigonometry  Operator=cos
  Trigonometric Function3 : Trigonometry
  WEarth : Constant  Value=WEarth
  AccZ Кориолис : Outport
  wires:
  Product5/1 -> Add1/2
  Add1/1 -> Product/3
  Product4/1 -> Add1/1
  2/1 -> Product/1
  Trigonometric Function2/1 -> Product4/2
  Trigonometric Function3/1 -> Product5/2
  WEarth/1 -> Product/2
  phi/1 -> Trigonometric Function2/1, Trigonometric Function3/1
  Product/1 -> Gain/1
  Gain/1 -> AccZ Кориолис/1
  VelY/1 -> Product4/1
  VelX/1 -> Product5/1

== system UAVIntegratedNavigationSystem/Блок модели динамики квадрокоптера + САУ/Упрощенная динамика БЛА /Простр. движение Ц.М. БПЛА (Геогр. СК)/Скорости БПЛА (Географ. СК)/dVz // dt/AccZ Относительное ==
  VelX : Inport
  VelY : Inport  Port=2
  VelZ : Inport  Port=3
  R : Inport  Port=4
  phi : Inport  Port=5
  Add : Sum  Inputs=+-
  Demux : Demux  Outputs=2
  Divide : Product  Inputs=*/
  Divide1 : Product  Inputs=*/
  Product1 : Product
  Product2 : Product
  Product3 : Product
  Trigonometric Function1 : Trigonometry  Operator=tan
  AccZ Относительное : Outport
  wires:
  R/1 -> Demux/1
  Demux/2 -> Divide1/2  "R2"
  Trigonometric Function1/1 -> Product3/2
  Divide1/1 -> Product3/1
  Product2/1 -> Divide1/1
  phi/1 -> Trigonometric Function1/1
  Product3/1 -> Add/1
  Add/1 -> AccZ Относительное/1
  Demux/1 -> Divide/2  "R1"
  Product1/1 -> Divide/1
  Divide/1 -> Add/2
  VelY/1 -> Product1/1
  VelZ/1 -> Product2/2, Product1/2
  VelX/1 -> Product2/1

== matlab function UAVIntegratedNavigationSystem/Subsystem/MATLAB Function1 ==
  data: SampleGNSSOff input; y output; SampleAINSOff input; INSGNSS input; INSAINS input
function y = fcn(SampleGNSSOff, SampleAINSOff, INSGNSS, INSAINS)
if (SampleGNSSOff < SampleAINSOff)
    y = INSGNSS;
elseif (SampleGNSSOff > SampleAINSOff)
    y = INSAINS;
else
    y = INSGNSS;
end

== matlab function UAVIntegratedNavigationSystem/Блок создания траектории движения БЛА/If Action Subsystem/Start Path Coordinate ==
  data: X output; Z output; t input; TAltitude input; NorthInit input; EastInit input
function [X, Z]  = fcn(t, TAltitude, NorthInit, EastInit)
if ((t>=0) && (t<3))
     X = NorthInit;
     Z = EastInit;
 elseif ((t>=3) && (t<15))  
     X = NorthInit;
     Z = EastInit;
 elseif ((t>=15) && (t<25))  
     X = NorthInit;
     Z = EastInit;
   elseif ((t>=25) && (t<30))  
     X = NorthInit;
     Z = EastInit;   
    elseif ((t>=30) && (t<35))  
     X = NorthInit;
     Z = EastInit;
    elseif ((t>=35) && (t<50))  
     X = NorthInit;
     Z = EastInit;
    elseif ((t>=50) && (t<65))  
     X = NorthInit;
     Z = EastInit; 
    elseif ((t>=65) && (t<75))  
     X = NorthInit;
     Z = EastInit; 
    elseif ((t>=75) && (t<85))  
     X = NorthInit;
     Z = EastInit;
    elseif ((t>=85) && (t<TAltitude))  
     X = NorthInit;
     Z = EastInit;
 else
     X = NorthInit;
     Z = EastInit;
end
